simulink model "tank_model_test_harness"  (R2025b)
settings: Solver=VariableStepAuto  StartTime=0.0  StopTime=84  MaxStep=1e-3  RelTol=1e-3
InitFcn:
  | fluid_constants;
undefined symbols (not defined in the file or in its folder): fluid, ts, ts2, valveFit
libraries: metux_library x2, eeGeneralControl x1
settings Model: Creator=karadeli  LastModifiedBy=karadeli

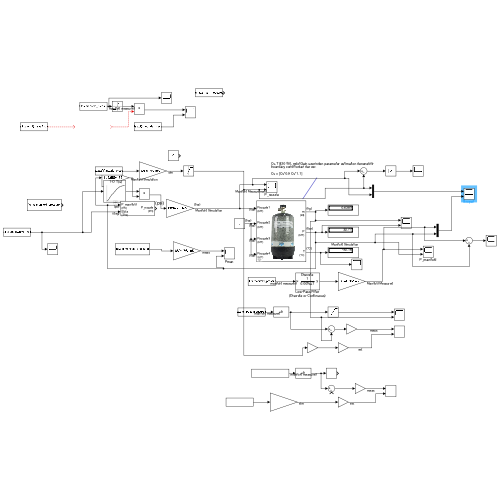
[thumbnail: Simulink's stored preview of the top-level diagram]
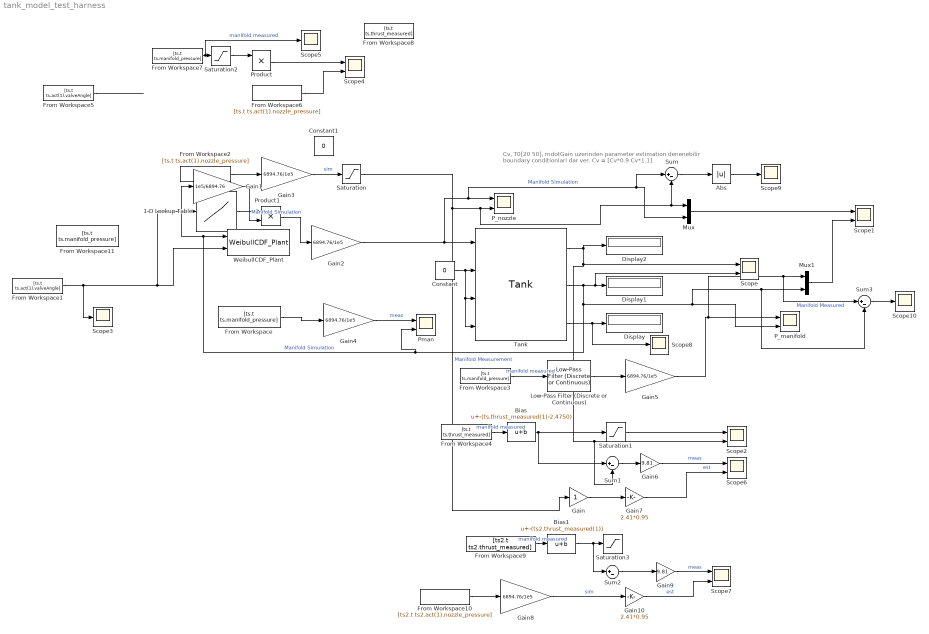
== system tank_model_test_harness ==
  note: Cv, T0[20 50], mdotGain uzerinden parameter estimation denenebilir
      | boundary conditionlari dar ver.
      |
      | Cv = [Cv*0.9 Cv*1.1]
  1-D Lookup Table : Lookup_n-D  NumberOfTableDimensions=1  BreakpointsForDimension1=valveFit.angles  Table=valveFit.pressureRatios  InterpMethod=Linear Lagrange  ExtrapMethod=Clip  InternalRulePriority=Speed  RndMeth=Simplest
  Abs : Abs  SaturateOnIntegerOverflow=off
  Bias : Bias  Bias=-(ts.thrust_measured(1)-2.4750)  SaturateOnIntegerOverflow=off
  Bias1 : Bias  Bias=-(ts2.thrust_measured(1))  SaturateOnIntegerOverflow=off
  Constant : Constant  Value=0
  Constant1 : Constant  Value=0
  Display : Display
  Display1 : Display
  Display2 : Display
  From Workspace{,3,7,11} (4 alike) : FromWorkspace  VariableName=[ts.t ts.manifold_pressure]
  From Workspace1 : FromWorkspace  VariableName=[ts.t ts.act(1).valveAngle]  SampleTime=1e-3
  From Workspace10 : FromWorkspace  VariableName=[ts2.t ts2.act(1).nozzle_pressure]
  From Workspace2 : FromWorkspace  VariableName=[ts.t ts.act(1).nozzle_pressure]
  From Workspace4 : FromWorkspace  VariableName=[ts.t ts.thrust_measured]
  From Workspace5 : FromWorkspace  VariableName=[ts.t ts.act(1).valveAngle]  SampleTime=1e-3
  From Workspace6 : FromWorkspace  VariableName=[ts.t ts.act(1).nozzle_pressure]
  From Workspace8 : FromWorkspace  VariableName=[ts.t ts.thrust_measured]
  From Workspace9 : FromWorkspace  VariableName=[ts2.t ts2.thrust_measured]
  Gain : Gain
  Gain1 : Gain  Gain=1e5/6894.76
  Gain10 : Gain  Gain=2.41*0.95
  Gain{2..5,8} (5 alike) : Gain  Gain=6894.76/1e5
  Gain6 : Gain  Gain=9.81
  Gain7 : Gain  Gain=2.41*0.95
  Gain9 : Gain  Gain=9.81
  Low-Pass Filter (Discrete or Continuous) : eeGeneralControl/Low-Pass Filter (Discrete or Continuous)  K=1  T=0.005  B=inf  A=-inf  init_option=Inherited from block input  x0=0  Ts=-1
  Mux : Mux  Inputs=2
  Mux1 : Mux  Inputs=2
  P_manifold : Scope  NumInputPorts=2
      settings: ActiveDisplayYMinimum=-33.344056032852549  ActiveDisplayYMaximum=300.09871862738441  DataLoggingVariableName=ScopeData3
  P_nozzle : Scope  NumInputPorts=2
      settings: ActiveDisplayYMinimum=-4.63385796317948  ActiveDisplayYMaximum=171.98365909728312
  Pman : Scope  NumInputPorts=2
      settings: ActiveDisplayYMinimum=-33.70781202058739  ActiveDisplayYMaximum=314.30167565734388  DataLoggingVariableName=ScopeData2
  Product : Product
  Product1 : Product
  Saturation : Saturate  UpperLimit=inf  LowerLimit=0
  Saturation1 : Saturate  UpperLimit=5  LowerLimit=-5
  Saturation2 : Saturate  UpperLimit=inf  LowerLimit=14
  Saturation3 : Saturate  UpperLimit=5  LowerLimit=-5
  Scope{,1..2,4,6..7} (6 alike) : Scope  NumInputPorts=2
      Scope settings: ActiveDisplayYMinimum=0.13872064426041808  ActiveDisplayYMaximum=2.9403225578934014
      Scope1 settings: ActiveDisplayYMinimum=-10.745198269472093  ActiveDisplayYMaximum=96.706784425248856  DataLoggingVariableName=ScopeData10
      Scope2 settings: ActiveDisplayYMinimum=-0.988842845917533  ActiveDisplayYMaximum=5.6654269828797261  DataLoggingVariableName=ScopeData4
      Scope4 settings: ActiveDisplayYMinimum=-295.87503789904423  ActiveDisplayYMaximum=2607.1112091805803  DataLoggingVariableName=ScopeData5
      Scope6 settings: ActiveDisplayYMinimum=-49.635178294774931  ActiveDisplayYMaximum=411.87244080603875  DataLoggingVariableName=ScopeData8
      Scope7 settings: ActiveDisplayYMinimum=50.093516413502357  ActiveDisplayYMaximum=124.92944595927354  DataLoggingVariableName=ScopeData9
  Scope{3,5,8..10} (5 alike) : Scope
      Scope10 settings: ActiveDisplayYMinimum=-3.2329259963643935  ActiveDisplayYMaximum=3.9698815108527867  DataLoggingVariableName=ScopeData13
      Scope3 settings: ActiveDisplayYMinimum=-136.46939630806412  ActiveDisplayYMaximum=1216.5365572720739  DataLoggingVariableName=ScopeData6
      Scope5 settings: ActiveDisplayYMinimum=13.961869344046818  ActiveDisplayYMaximum=108.78512346132811  DataLoggingVariableName=ScopeData7
      Scope8 settings: ActiveDisplayYMinimum=-1  ActiveDisplayYMaximum=1  DataLoggingVariableName=ScopeData11
      Scope9 settings: ActiveDisplayYMinimum=-2.7435802015589852  ActiveDisplayYMaximum=24.692221814030869  DataLoggingVariableName=ScopeData12
  Sum{,1..3} (4 alike) : Sum  Inputs=|+-
  Tank : metux_library/Tank  P0=ts.manifold_pressure(1)*6894.76/1e5  T0=36  mdotGain=fluid.mdotGain*1.3  V=fluid.V  R=fluid.R  Cv=fluid.Cv  Patm=fluid.Patm
  WeibullCDF_Plant : metux_library/WeibullCDF_Plant  L=0.7772  tau=519.6652  n=1.5198
  wires:
  Tank/1 -> Display2/1, Sum1/2, Scope2/2, Scope/1
  From Workspace2/1 -> Gain3/1
  Tank/3 -> Scope8/1, Display/1
  Tank/2 -> Mux1/2, Sum3/2, P_manifold/2, Gain1/1, WeibullCDF_Plant/1, Pman/2, Scope/2, Display1/1  "Manifold Simulation"
  From Workspace1/1 -> 1-D Lookup Table/1, WeibullCDF_Plant/2, Scope3/1
  From Workspace/1 -> Gain4/1
  Gain4/1 -> Pman/1  "meas"
  Constant/1 -> Tank/3, Tank/4, Tank/2
  From Workspace3/1 -> Low-Pass Filter (Discrete or Continuous)/1  "manifold measured"
  Gain5/1 -> Sum3/1, Mux1/1, P_manifold/1  "Manifold Measured"
  Low-Pass Filter (Discrete or Continuous)/1 -> Gain5/1
  Gain2/1 -> Tank/1, Sum/1, Mux/2, P_nozzle/1  "Manifold Simulation"
  From Workspace4/1 -> Bias/1  "manifold measured"
  Gain3/1 -> Saturation/1  "sim"
  Saturation/1 -> Sum/2, Mux/1, P_nozzle/2, Gain/1  "Manifold Measurement"
  From Workspace5/1 -> ?
  From Workspace7/1 -> Scope5/1, Saturation2/1  "manifold measured"
  Saturation2/1 -> Product/1
  ? -> Product/2
  Product/1 -> Scope4/1
  From Workspace6/1 -> Scope4/2
  Saturation1/1 -> Scope2/1
  Sum1/1 -> Gain6/1
  Bias/1 -> Sum1/1, Saturation1/1
  Gain/1 -> Gain7/1
  Gain6/1 -> Scope6/1  "meas"
  Gain7/1 -> Scope6/2  "est"
  From Workspace9/1 -> Bias1/1  "manifold measured"
  Bias1/1 -> Sum2/1, Saturation3/1
  From Workspace10/1 -> Gain8/1
  Sum2/1 -> Gain9/1
  Gain9/1 -> Scope7/1  "meas"
  Gain8/1 -> Gain10/1  "sim"
  Gain10/1 -> Scope7/2  "est"
  Mux/1 -> Scope1/1
  Mux1/1 -> Scope1/2
  Sum/1 -> Abs/1
  Abs/1 -> Scope9/1
  1-D Lookup Table/1 -> Product1/1
  Product1/1 -> Gain2/1
  Gain1/1 -> Product1/2  "Manifold Simulation"
  Sum3/1 -> Scope10/1
